simulink model "make_simulation"  (R2018a)
settings: Solver=VariableStepAuto  StartTime=0.0  StopTime=200  RelTol=1e-3
InitFcn:
  | init
libraries: simulink x1
settings Model: Creator=kyniu  LastModifiedBy=kuba

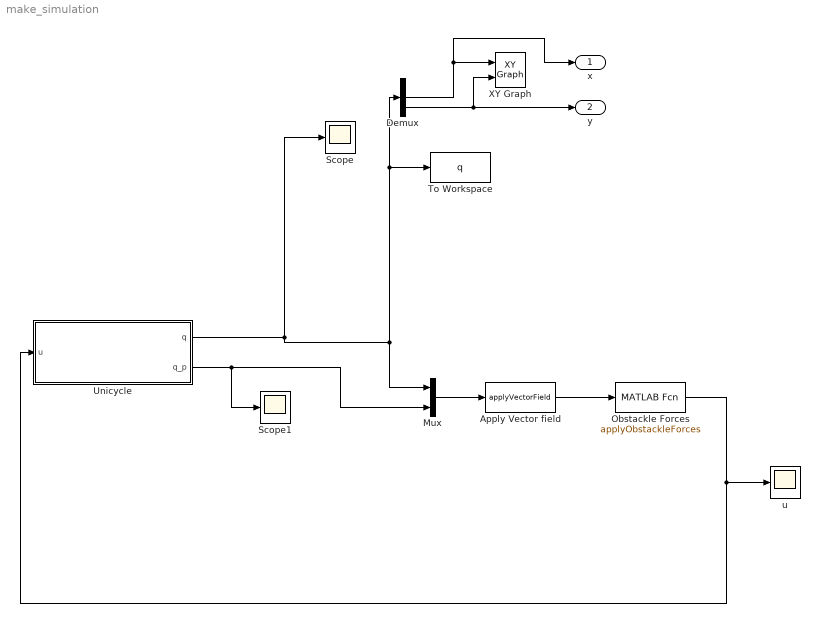
== system make_simulation ==
  "Apply Vector field " : MATLABFcn  MATLABFcn=applyVectorField
  Demux : Demux  Outputs=3
  Mux : Mux  Inputs=2
  "Obstackle Forces " : MATLABFcn  MATLABFcn=applyObstackleForces
  Scope : Scope
  Scope1 : Scope
  To Workspace : ToWorkspace  VariableName=q  SaveFormat=Timeseries  SampleTime=-1
  Unicycle : Subsystem
  XY Graph : simulink/Sinks/XY Graph  xmin=0  xmax=100  ymin=0  ymax=100  st=-1
  u : Scope
  x : Outport
  y : Outport  Port=2
  wires:
  Unicycle/2(q_p) -> Mux/2, Scope1/1
  Unicycle/1(q) -> Demux/1, To Workspace/1, Mux/1, Scope/1
  Demux/2 -> x/1, XY Graph/1
  Demux/3 -> y/1, XY Graph/2
  Mux/1 -> "Apply Vector field "/1
  "Obstackle Forces "/1 -> Unicycle/1(u), u/1
  "Apply Vector field "/1 -> "Obstackle Forces "/1

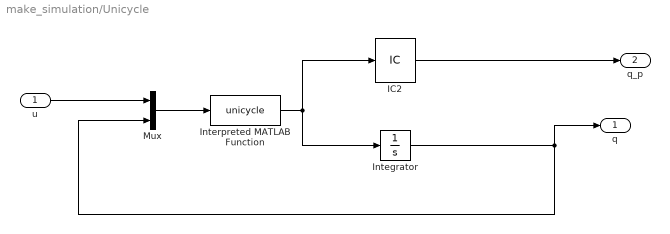
== system make_simulation/Unicycle ==
  u : Inport
  IC2 : InitialCondition  Value=[0;0;0]
  Integrator : Integrator  InitialCondition=[pi/2; 20;0]
  Interpreted MATLAB Function : MATLABFcn  MATLABFcn=unicycle
  Mux : Mux  Inputs=2
  q : Outport
  q_p : Outport  Port=2
  wires:
  Integrator/1 -> q/1, Mux/2
  IC2/1 -> q_p/1
  Mux/1 -> Interpreted MATLAB Function/1
  Interpreted MATLAB Function/1 -> Integrator/1, IC2/1
  u/1 -> Mux/1
